simulink model "sampleModel1823"  (R2023a)
settings: Solver=VariableStepAuto  StartTime=0.0  StopTime=10.0  RelTol=1e-3
libraries: hdlsllib x3, simulink x1
settings Model: Creator=user1  LastModifiedBy=user1

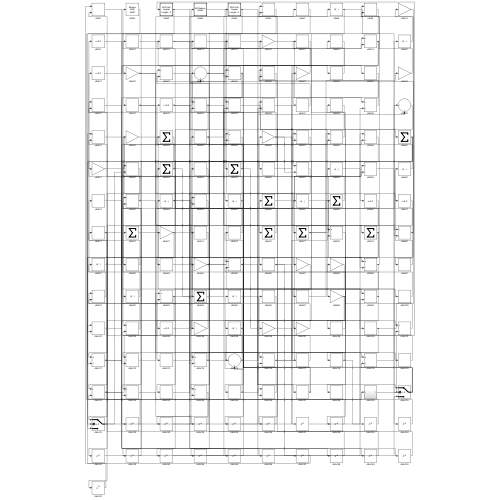
[thumbnail: Simulink's stored preview of the top-level diagram]
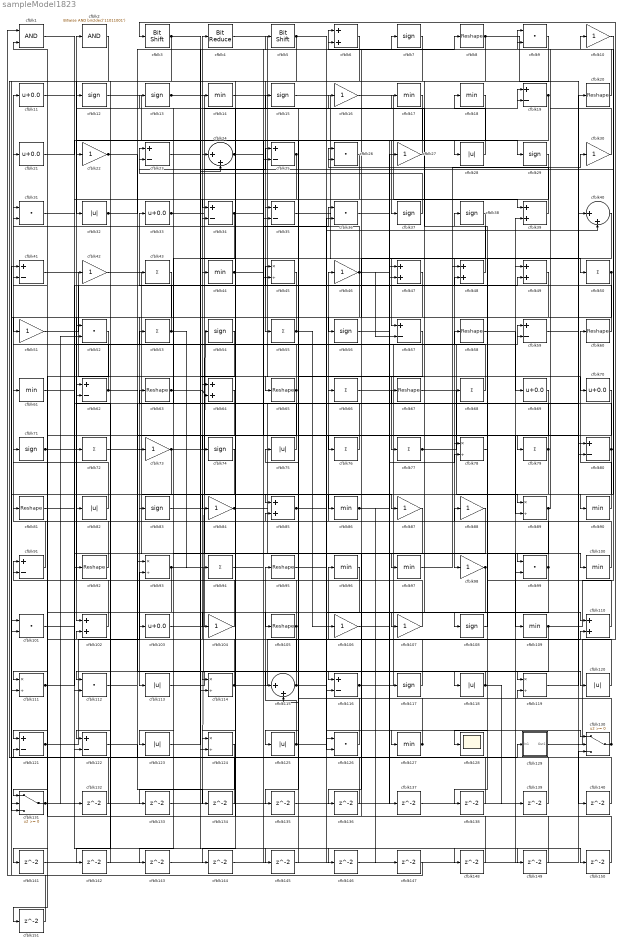
== system sampleModel1823 ==
  cfblk1 : Logic  AllPortsSameDT=off  OutDataTypeStr=boolean
  cfblk{10,16,22,27,30,42,46,51,73,84,87..88,98,104,106..107} (16 alike) : Gain
  cfblk{14,17..18,44,61,86,90,96..97,100,109,127} (12 alike) : MinMax
  cfblk{9,26,31,36,52,99,101,112,126} (9 alike) : DotProduct  OutDataTypeStr=Inherit: Inherit via internal rule
  cfblk{6,39,47..49,64,85,102,110} (9 alike) : Sum
  cfblk{11,21,33,69..70,103} (6 alike) : Bias  Bias=0.0  SaturateOnIntegerOverflow=off
  cfblk{8,20,58,60,63,65,67,81,92,95,105} (11 alike) : Reshape
  cfblk{7,12..13,15,29,37..38,54,56,71,74,83,108,117} (14 alike) : Signum
  cfblk{45,78,89,93,111,114,119,124} (8 alike) : Product  Inputs=*/  RndMeth=Zero  SaturateOnIntegerOverflow=on
  cfblk{28,32,75,82,113,118,120,123,125} (9 alike) : Abs  SaturateOnIntegerOverflow=off
  cfblk115 : Sum  Inputs=|++
  cfblk{19,23,25,34..35,41,57,59,62,80,91,116,121..122} (14 alike) : Sum  Inputs=+-
  cfblk128 : Scope
  cfblk129 : Subsystem
      settings: LibrarySourceBlock=|
      | hdlsllib/Ports &
      | Subsystems/Subsystem
  cfblk130 : Switch  SaturateOnIntegerOverflow=off  InputSameDT=off
  cfblk131 : Switch  SaturateOnIntegerOverflow=off  InputSameDT=off
  cfblk{132..151} (20 alike) : Delay  SampleTime=1
  cfblk2 : simulink/Logic and Bit Operations/Bitwise Operator  logicop=AND  UseBitMask=on  BitMask=bin2dec('11011001')  BitMaskRealWorld=Stored Integer
      settings: LibrarySourceBlock=|
      | hdlsllib/Logic and Bit
      | Operations/Bitwise
      | Operator
  cfblk24 : Sum  Inputs=|++
  cfblk3 : hdlsllib/Logic and Bit Operations/Bit Shift  mode=Shift Left Logical  N=0
  cfblk4 : hdlsllib/Logic and Bit Operations/Bit Reduce  mode=AND
  cfblk40 : Sum  Inputs=|++
  cfblk{43,50,53,55,66,68,72,76..77,79,94} (11 alike) : Sum  Inputs=+
  cfblk5 : hdlsllib/Logic and Bit Operations/Bit Shift  mode=Shift Left Logical  N=0
  wires:
  cfblk100/1 -> cfblk46/1
  cfblk73/1 -> cfblk86/1, cfblk131/3
  cfblk116/1 -> cfblk59/1, cfblk78/2
  cfblk35/1 -> cfblk98/1
  cfblk109/1 -> cfblk23/1, cfblk115/2
  cfblk65/1 -> cfblk102/1, cfblk31/2
  cfblk16/1 -> cfblk39/1
  cfblk114/1 -> cfblk4/1, cfblk36/2
  cfblk42/1 -> cfblk87/1
  cfblk68/1 -> cfblk11/1
  cfblk15/1 -> cfblk57/1
  cfblk78/1 -> cfblk108/1
  cfblk93/1 -> cfblk19/1, cfblk112/2
  cfblk43/1 -> cfblk113/1
  cfblk41/1 -> cfblk65/1
  cfblk20/1 -> cfblk6/1
  cfblk129/1(Out1) -> cfblk3/1
  cfblk14/1 -> cfblk77/1
  cfblk83/1 -> cfblk99/1
  cfblk91/1 -> cfblk21/1
  cfblk9/1 -> cfblk55/1
  cfblk125/1 -> cfblk95/1, cfblk40/2
  cfblk33/1 -> cfblk25/1, cfblk120/1
  cfblk57/1 -> cfblk105/1
  cfblk2/1 -> cfblk129/1(In1)
  cfblk92/1 -> cfblk2/1
  cfblk47/1 -> cfblk123/1
  cfblk70/1 -> cfblk125/1
  cfblk121/1 -> cfblk93/2, cfblk148/1
  cfblk130/1 -> cfblk63/1, cfblk75/1, cfblk119/2
  cfblk107/1 -> cfblk42/1
  cfblk77/1 -> cfblk59/2, cfblk30/1
  cfblk118/1 -> cfblk112/1, cfblk139/1
  cfblk26/1 -> cfblk35/1
  cfblk13/1 -> cfblk19/2, cfblk149/1
  cfblk131/1 -> cfblk54/1, cfblk52/2
  cfblk127/1 -> cfblk44/1, cfblk31/1
  cfblk58/1 -> cfblk69/1
  cfblk67/1 -> cfblk89/1
  cfblk24/1 -> cfblk16/1, cfblk80/2
  cfblk49/1 -> cfblk82/1
  cfblk82/1 -> cfblk61/1
  cfblk12/1 -> cfblk24/2
  cfblk90/1 -> cfblk60/1
  cfblk66/1 -> cfblk49/1
  cfblk18/1 -> cfblk47/2
  cfblk72/1 -> cfblk109/1
  cfblk75/1 -> cfblk64/1
  cfblk103/1 -> cfblk20/1
  cfblk17/1 -> cfblk25/2
  cfblk6/1 -> cfblk32/1
  cfblk89/1 -> cfblk9/1, cfblk138/1
  cfblk108/1 -> cfblk38/1
  cfblk8/1 -> cfblk80/1, cfblk97/1
  cfblk51/1 -> cfblk49/2
  cfblk97/1 -> cfblk68/1
  cfblk60/1 -> cfblk33/1
  cfblk69/1 -> cfblk89/2
  cfblk29/1 -> cfblk104/1
  cfblk46/1 -> cfblk14/1, cfblk79/1, cfblk73/1, cfblk57/2
  cfblk10/1 -> cfblk90/1
  cfblk110/1 -> cfblk88/1
  cfblk84/1 -> cfblk48/1, cfblk130/2
  cfblk86/1 -> cfblk119/1, cfblk147/1
  cfblk37/1 -> cfblk23/2
  cfblk79/1 -> cfblk45/1, cfblk128/1, cfblk114/1
  cfblk53/1 -> cfblk43/1, cfblk94/1
  cfblk117/1 -> cfblk96/1
  cfblk80/1 -> cfblk10/1, cfblk111/2, cfblk13/1
  cfblk4/1 -> cfblk37/1
  cfblk32/1 -> cfblk8/1, cfblk74/1
  cfblk63/1 -> cfblk64/2, cfblk146/1
  cfblk120/1 -> cfblk71/1
  cfblk126/1 -> cfblk12/1
  cfblk1/1 -> cfblk92/1
  cfblk7/1 -> cfblk22/1
  cfblk30/1 -> cfblk9/2
  cfblk111/1 -> cfblk58/1, cfblk145/1
  cfblk102/1 -> cfblk91/1
  cfblk27/1 -> cfblk15/1
  cfblk56/1 -> cfblk27/1
  cfblk64/1 -> cfblk111/1
  cfblk115/1 -> cfblk62/1, cfblk110/2
  cfblk45/1 -> cfblk124/1
  cfblk22/1 -> cfblk70/1, cfblk76/1
  cfblk119/1 -> cfblk40/1
  cfblk36/1 -> cfblk117/1
  cfblk112/1 -> cfblk67/1
  cfblk21/1 -> cfblk28/1
  cfblk113/1 -> cfblk116/1
  cfblk98/1 -> cfblk103/1, cfblk115/1
  cfblk104/1 -> cfblk41/2
  cfblk94/1 -> cfblk36/1
  cfblk55/1 -> cfblk51/1, cfblk106/1
  cfblk39/1 -> cfblk26/1
  cfblk48/1 -> cfblk17/1
  cfblk71/1 -> cfblk121/1, cfblk72/1
  cfblk31/1 -> cfblk100/1
  cfblk95/1 -> cfblk110/1
  cfblk101/1 -> cfblk66/1
  cfblk38/1 -> cfblk56/1
  cfblk85/1 -> cfblk127/1, cfblk135/1
  cfblk105/1 -> cfblk62/2, cfblk144/1
  cfblk54/1 -> cfblk124/2
  cfblk19/1 -> cfblk122/1, cfblk85/1
  cfblk3/1 -> cfblk101/2, cfblk29/1
  cfblk76/1 -> cfblk53/1
  cfblk5/1 -> cfblk34/1, cfblk130/1
  cfblk50/1 -> cfblk131/2, cfblk107/1, cfblk142/1
  cfblk34/1 -> cfblk83/1, cfblk78/1
  cfblk62/1 -> cfblk52/1, cfblk114/2
  cfblk99/1 -> cfblk81/1, cfblk126/2
  cfblk28/1 -> cfblk18/1
  cfblk44/1 -> cfblk7/1, cfblk84/1
  cfblk25/1 -> cfblk45/2, cfblk122/2
  cfblk123/1 -> cfblk5/1
  cfblk81/1 -> cfblk48/2
  cfblk40/1 -> cfblk118/1
  cfblk23/1 -> cfblk50/1
  cfblk96/1 -> cfblk131/1
  cfblk61/1 -> cfblk132/1
  cfblk132/1 -> cfblk101/1
  cfblk124/1 -> cfblk133/1
  cfblk133/1 -> cfblk47/1
  cfblk122/1 -> cfblk134/1
  cfblk134/1 -> cfblk91/2
  cfblk135/1 -> cfblk126/1
  cfblk88/1 -> cfblk136/1
  cfblk136/1 -> cfblk34/2
  cfblk106/1 -> cfblk137/1
  cfblk137/1 -> cfblk99/2
  cfblk138/1 -> cfblk121/2
  cfblk139/1 -> cfblk6/2
  cfblk59/1 -> cfblk140/1
  cfblk140/1 -> cfblk93/1
  cfblk52/1 -> cfblk141/1
  cfblk141/1 -> cfblk39/2
  cfblk142/1 -> cfblk102/2
  cfblk87/1 -> cfblk143/1
  cfblk143/1 -> cfblk35/2
  cfblk144/1 -> cfblk116/2
  cfblk145/1 -> cfblk85/2
  cfblk146/1 -> cfblk130/3
  cfblk147/1 -> cfblk1/1
  cfblk148/1 -> cfblk26/2
  cfblk149/1 -> cfblk1/2
  cfblk11/1 -> cfblk150/1
  cfblk150/1 -> cfblk24/1
  cfblk74/1 -> cfblk151/1
  cfblk151/1 -> cfblk41/1

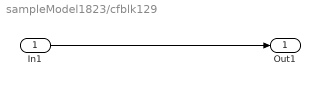
== system sampleModel1823/cfblk129 ==
  In1 : Inport
  Out1 : Outport
  wires:
  In1/1 -> Out1/1
